simulink model "exact_linearization_new"  (R2021b)
settings: Solver=ode45  StartTime=0.0  StopTime=100.0  RelTol=1e-10
values from neighbouring files (symbols this model uses):
  G = 9.81    [edda.m]
  K0 = 1    [edda.m]
  K1 = 1    [edda.m]
  O1 = 3.1    [edda.m]
  O2 = 9.5    [edda.m]
  O3 = 0.24    [edda.m]
  O4 = 0.77    [edda.m]
settings Model: Creator=mbober  LastModifiedBy=mbober
settings DebuggingCC: UnderSpecifiedDimensionMsg=error

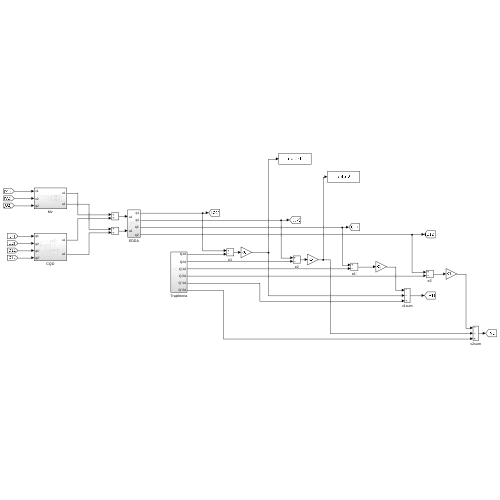
[thumbnail: Simulink's stored preview of the top-level diagram]
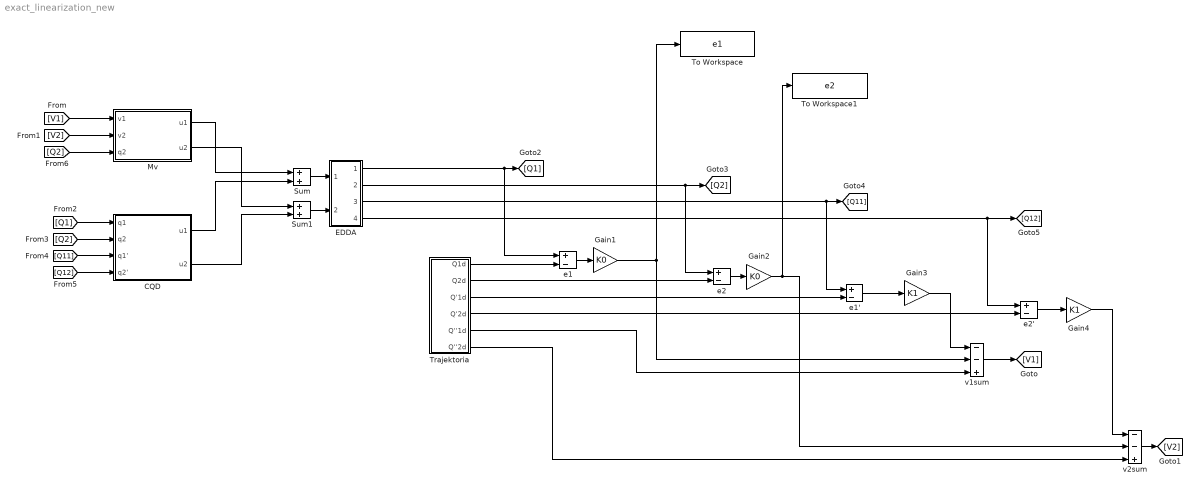
== system exact_linearization_new ==
  CQD : Subsystem
  EDDA : Subsystem
  Gain1 : Gain  Gain=K0
  Gain2 : Gain  Gain=K0
  Gain3 : Gain  Gain=K1
  Gain4 : Gain  Gain=K1
  Mv : Subsystem
  Sum : Sum
  Sum1 : Sum
  To Workspace : ToWorkspace  VariableName=e1  SampleTime=-1
  To Workspace1 : ToWorkspace  VariableName=e2  SampleTime=-1
  Trajektoria : Subsystem
  e1 : Sum  Inputs=+-
  e1' : Sum  Inputs=+-
  e2 : Sum  Inputs=+-
  e2' : Sum  Inputs=+-
  v1sum : Sum  Inputs=--+
  v2sum : Sum  Inputs=--+
  wires:
  Trajektoria/1(Q1d) -> e1/2
  EDDA/1(q1) -> [Q1], e1/1
  EDDA/2(q2) -> [Q2], e2/1
  Trajektoria/2(Q2d) -> e2/2
  EDDA/3(q1') -> [Q11], e1'/1
  Trajektoria/3(Q'1d) -> e1'/2
  EDDA/4(q2') -> e2'/1, [Q12]
  Trajektoria/4(Q'2d) -> e2'/2
  e1/1 -> Gain1/1
  e2/1 -> Gain2/1
  e1'/1 -> Gain3/1
  e2'/1 -> Gain4/1
  Gain3/1 -> v1sum/1
  Gain1/1 -> To Workspace/1, v1sum/2
  Gain4/1 -> v2sum/1
  Gain2/1 -> To Workspace1/1, v2sum/2
  Trajektoria/5(Q''1d) -> v1sum/3
  Trajektoria/6(Q''2d) -> v2sum/3
  v1sum/1 -> [V1]
  v2sum/1 -> [V2]
  [V1] -> Mv/1(v1)
  [V2] -> Mv/2(v2)
  [Q11] -> CQD/3(q1')
  [Q12] -> CQD/4(q2')
  [Q2] -> CQD/2(q2)
  [Q1] -> CQD/1(q1)
  [Q2] -> Mv/3(q2)
  Sum/1 -> EDDA/1(u1)
  Sum1/1 -> EDDA/2(u2)
  CQD/2(u2) -> Sum1/2
  Mv/2(u2) -> Sum1/1
  CQD/1(u1) -> Sum/2
  Mv/1(u1) -> Sum/1

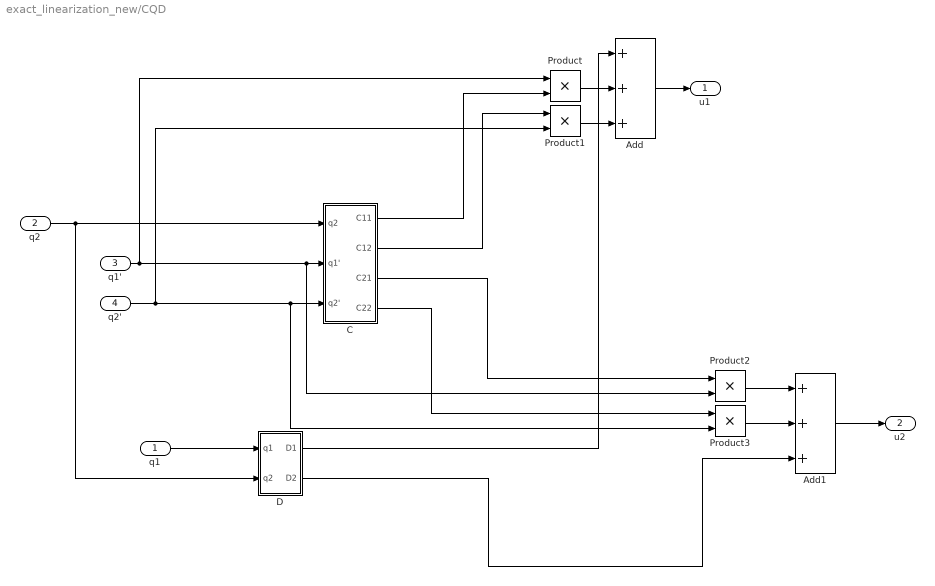
== system exact_linearization_new/CQD ==
  q1 : Inport
  q2 : Inport  Port=2
  q1' : Inport  Port=3
  q2' : Inport  Port=4
  Add : Sum  Inputs=+++
  Add1 : Sum  Inputs=+++
  C : Subsystem
  D : Subsystem
  Product{,1..3} (4 alike) : Product
  u1 : Outport
  u2 : Outport  Port=2
  wires:
  q2'/1 -> Product1/2, Product3/2, C/3(q2')
  q1'/1 -> Product2/2, C/2(q1'), Product/1
  q1/1 -> D/1(q1)
  q2/1 -> C/1(q2), D/2(q2)
  C/1(C11) -> Product/2
  C/2(C12) -> Product1/1
  Product/1 -> Add/2
  Product1/1 -> Add/3
  D/1(D1) -> Add/1
  Product3/1 -> Add1/2
  Product2/1 -> Add1/1
  D/2(D2) -> Add1/3
  C/3(C21) -> Product2/1
  C/4(C22) -> Product3/1
  Add/1 -> u1/1
  Add1/1 -> u2/1

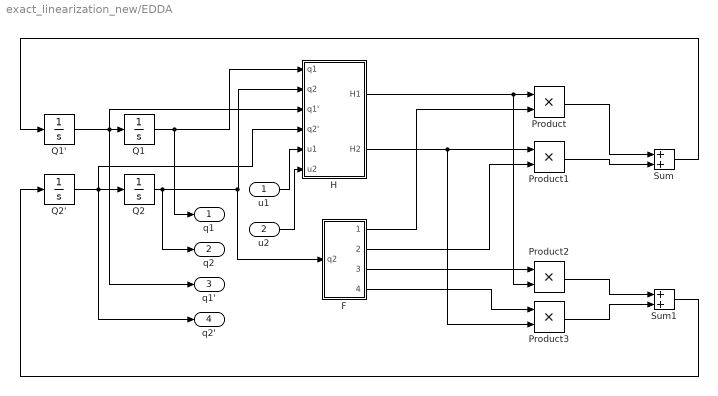
== system exact_linearization_new/EDDA ==
  u1 : Inport
  u2 : Inport  Port=2
  F : Subsystem
  H : Subsystem
  Product{,1..3} (4 alike) : Product
  Q1 : Integrator
  Q1' : Integrator
  Q2 : Integrator
  Q2' : Integrator
  Sum : Sum
  Sum1 : Sum
  q1 : Outport
  q2 : Outport  Port=2
  q1' : Outport  Port=3
  q2' : Outport  Port=4
  wires:
  Sum/1 -> Q1'/1
  F/3(F21) -> Product2/1
  u1/1 -> H/5(u1)
  Q2/1 -> q2/1, F/1(q2), H/2(q2)
  F/1(F11) -> Product/2
  Q1'/1 -> q1'/1, H/3(q1'), Q1/1
  Product1/1 -> Sum/2
  Q1/1 -> q1/1, H/1(q1)
  Q2'/1 -> q2'/1, H/4(q2'), Q2/1
  H/2(H2) -> Product3/2, Product1/1
  F/2(F12) -> Product1/2
  Sum1/1 -> Q2'/1
  u2/1 -> H/6(u2)
  H/1(H1) -> Product2/2, Product/1
  Product/1 -> Sum/1
  Product2/1 -> Sum1/1
  Product3/1 -> Sum1/2
  F/4(F22) -> Product3/1

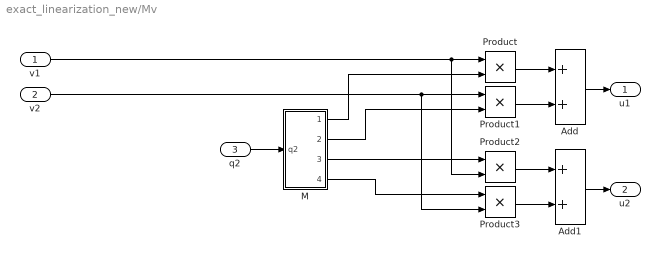
== system exact_linearization_new/Mv ==
  v1 : Inport
  v2 : Inport  Port=2
  q2 : Inport  Port=3
  Add : Sum
  Add1 : Sum
  M : Subsystem
  Product{,1..3} (4 alike) : Product
  u1 : Outport
  u2 : Outport  Port=2
  wires:
  q2/1 -> M/1(q2)
  Add/1 -> u1/1
  M/1(M11) -> Product/2
  v1/1 -> Product2/2, Product/1
  M/2(M12) -> Product1/2
  v2/1 -> Product3/2, Product1/1
  M/3(M21) -> Product2/1
  M/4(M22) -> Product3/1
  Product1/1 -> Add/2
  Product/1 -> Add/1
  Product2/1 -> Add1/1
  Product3/1 -> Add1/2
  Add1/1 -> u2/1

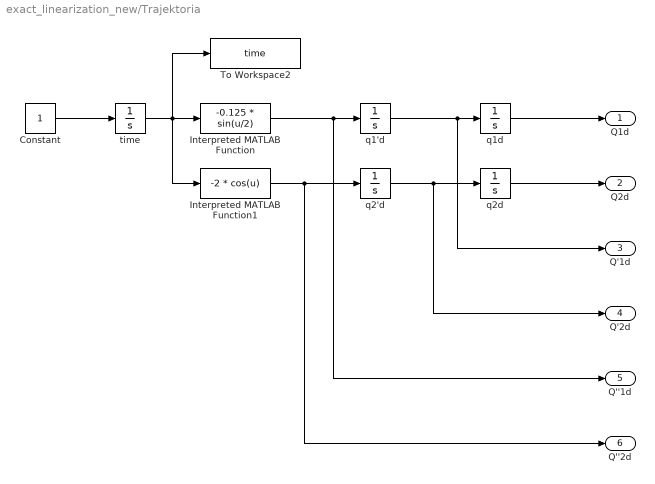
== system exact_linearization_new/Trajektoria ==
  Constant : Constant
  Interpreted MATLAB Function : MATLABFcn  MATLABFcn=-0.125 * sin(u/2)
  Interpreted MATLAB Function1 : MATLABFcn  MATLABFcn=-2 * cos(u)
  To Workspace2 : ToWorkspace  VariableName=time  SampleTime=-1
  q1'd : Integrator  InitialCondition=0.25
  q1d : Integrator
  q2'd : Integrator
  q2d : Integrator  InitialCondition=2
  time : Integrator
  Q1d : Outport
  Q2d : Outport  Port=2
  Q'1d : Outport  Port=3
  Q'2d : Outport  Port=4
  Q''1d : Outport  Port=5
  Q''2d : Outport  Port=6
  wires:
  q1d/1 -> Q1d/1
  Interpreted MATLAB Function/1 -> Q''1d/1, q1'd/1
  q2d/1 -> Q2d/1
  Interpreted MATLAB Function1/1 -> Q''2d/1, q2'd/1
  q1'd/1 -> Q'1d/1, q1d/1
  q2'd/1 -> Q'2d/1, q2d/1
  Constant/1 -> time/1
  time/1 -> Interpreted MATLAB Function1/1, To Workspace2/1, Interpreted MATLAB Function/1

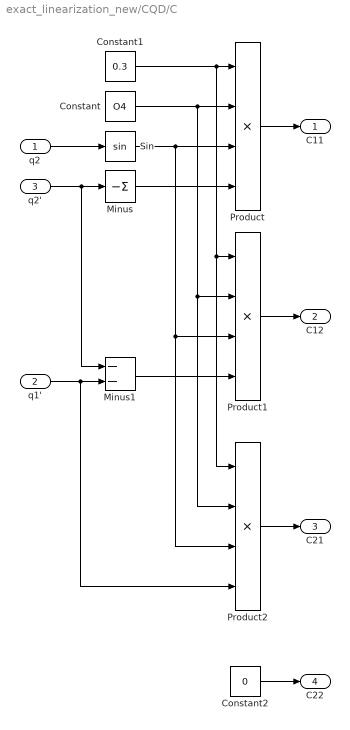
== system exact_linearization_new/CQD/C ==
  q2 : Inport
  q1' : Inport  Port=2
  q2' : Inport  Port=3
  Constant : Constant  Value=O4
  Constant1 : Constant  Value=0.3
  Constant2 : Constant  Value=0
  Minus : Sum  Inputs=-
  Minus1 : Sum  Inputs=--
  Product : Product  Inputs=4
  Product1 : Product  Inputs=4
  Product2 : Product  Inputs=4
  Sin : Trigonometry
  C11 : Outport
  C12 : Outport  Port=2
  C21 : Outport  Port=3
  C22 : Outport  Port=4
  wires:
  q2/1 -> Sin/1
  Sin/1 -> Product2/3, Product1/3, Product/3
  Constant/1 -> Product2/2, Product1/2, Product/2
  Constant1/1 -> Product2/1, Product1/1, Product/1
  Product/1 -> C11/1
  Minus/1 -> Product/4
  q2'/1 -> Minus1/1, Minus/1
  Minus1/1 -> Product1/4
  q1'/1 -> Product2/4, Minus1/2
  Product1/1 -> C12/1
  Product2/1 -> C21/1
  Constant2/1 -> C22/1

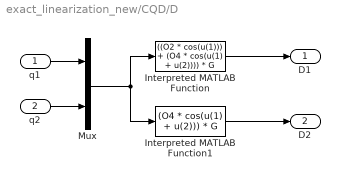
== system exact_linearization_new/CQD/D ==
  q1 : Inport
  q2 : Inport  Port=2
  Interpreted MATLAB Function : MATLABFcn  MATLABFcn=((O2 * cos(u(1))) + (O4 * cos(u(1) + u(2)))) * G
  Interpreted MATLAB Function1 : MATLABFcn  MATLABFcn=(O4 * cos(u(1) + u(2))) * G
  Mux : Mux  Inputs=2
  D1 : Outport
  D2 : Outport  Port=2
  wires:
  Interpreted MATLAB Function1/1 -> D2/1
  q1/1 -> Mux/1
  Mux/1 -> Interpreted MATLAB Function/1, Interpreted MATLAB Function1/1
  q2/1 -> Mux/2
  Interpreted MATLAB Function/1 -> D1/1

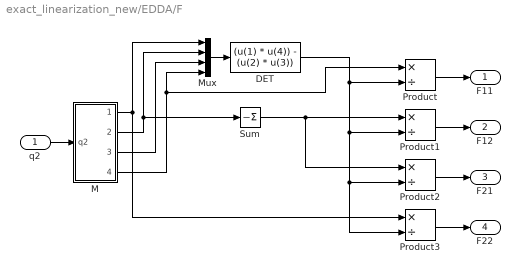
== system exact_linearization_new/EDDA/F ==
  q2 : Inport
  DET : MATLABFcn  MATLABFcn=(u(1) * u(4)) - (u(2) * u(3))  OutputDimensions=1
  M : Subsystem
  Mux : Mux
  Product{,1..3} (4 alike) : Product  Inputs=*/
  Sum : Sum  Inputs=-
  F11 : Outport
  F12 : Outport  Port=2
  F21 : Outport  Port=3
  F22 : Outport  Port=4
  wires:
  Product1/1 -> F12/1
  Mux/1 -> DET/1
  Product2/1 -> F21/1
  Product/1 -> F11/1
  M/2(M12) -> Mux/2, Sum/1
  M/1(M11) -> Product3/1, Mux/1
  M/4(M22) -> Product/1, Mux/4
  DET/1 -> Product/2, Product2/2, Product3/2, Product1/2
  Product3/1 -> F22/1
  q2/1 -> M/1(q2)
  M/3(M21) -> Mux/3
  Sum/1 -> Product2/1, Product1/1

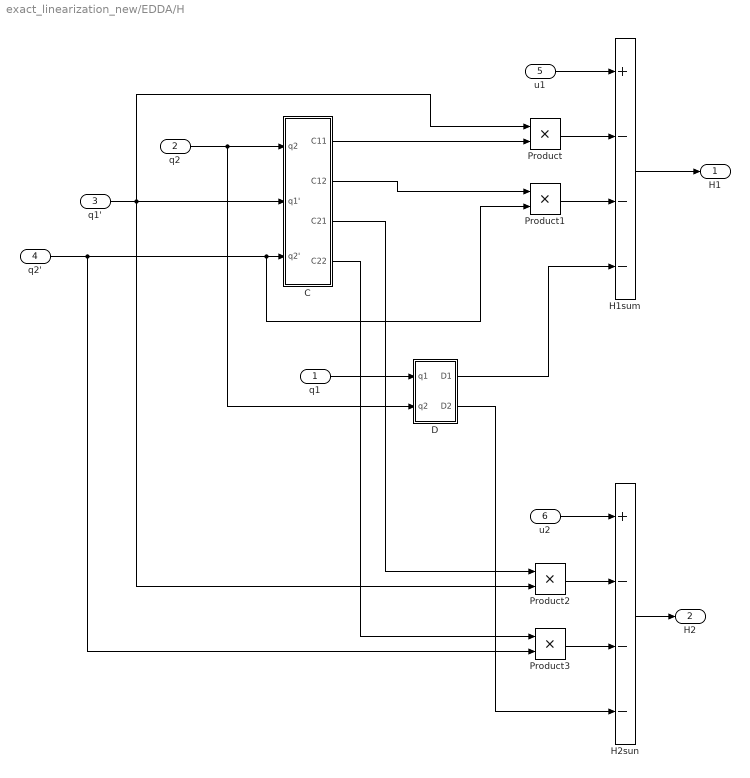
== system exact_linearization_new/EDDA/H ==
  q1 : Inport
  q2 : Inport  Port=2
  q1' : Inport  Port=3
  q2' : Inport  Port=4
  u1 : Inport  Port=5
  u2 : Inport  Port=6
  C : Subsystem
  D : Subsystem
  H1sum : Sum  Inputs=+---  OutMin=[1]  OutMax=[1]
  H2sun : Sum  Inputs=+---
  Product{,1..3} (4 alike) : Product
  H1 : Outport
  H2 : Outport  Port=2
  wires:
  Product2/1 -> H2sun/2
  C/4(C22) -> Product3/1
  Product1/1 -> H1sum/3
  D/1(D1) -> H1sum/4
  q1'/1 -> C/2(q1'), Product/1, Product2/2
  Product/1 -> H1sum/2
  q1/1 -> D/1(q1)
  q2/1 -> D/2(q2), C/1(q2)
  C/1(C11) -> Product/2
  u2/1 -> H2sun/1
  C/3(C21) -> Product2/1
  C/2(C12) -> Product1/1
  H1sum/1 -> H1/1
  D/2(D2) -> H2sun/4
  H2sun/1 -> H2/1
  Product3/1 -> H2sun/3
  q2'/1 -> Product1/2, C/3(q2'), Product3/2
  u1/1 -> H1sum/1

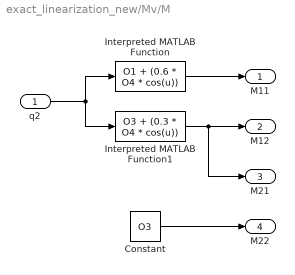
== system exact_linearization_new/Mv/M ==
  q2 : Inport
  Constant : Constant  Value=O3
  Interpreted MATLAB Function : MATLABFcn  MATLABFcn=O1 + (0.6 * O4 * cos(u))
  Interpreted MATLAB Function1 : MATLABFcn  MATLABFcn=O3 + (0.3 * O4 * cos(u))
  M11 : Outport
  M12 : Outport  Port=2
  M21 : Outport  Port=3
  M22 : Outport  Port=4
  wires:
  Interpreted MATLAB Function/1 -> M11/1
  q2/1 -> Interpreted MATLAB Function1/1, Interpreted MATLAB Function/1
  Interpreted MATLAB Function1/1 -> M21/1, M12/1
  Constant/1 -> M22/1

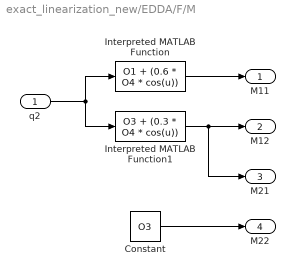
== system exact_linearization_new/EDDA/F/M ==
  q2 : Inport
  Constant : Constant  Value=O3
  Interpreted MATLAB Function : MATLABFcn  MATLABFcn=O1 + (0.6 * O4 * cos(u))
  Interpreted MATLAB Function1 : MATLABFcn  MATLABFcn=O3 + (0.3 * O4 * cos(u))
  M11 : Outport
  M12 : Outport  Port=2
  M21 : Outport  Port=3
  M22 : Outport  Port=4
  wires:
  Interpreted MATLAB Function/1 -> M11/1
  q2/1 -> Interpreted MATLAB Function1/1, Interpreted MATLAB Function/1
  Interpreted MATLAB Function1/1 -> M21/1, M12/1
  Constant/1 -> M22/1

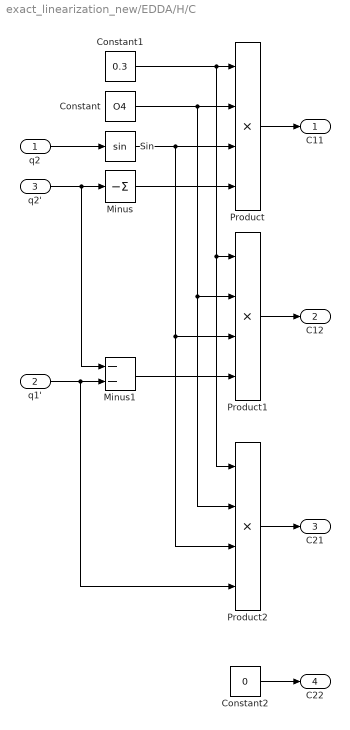
== system exact_linearization_new/EDDA/H/C ==
  q2 : Inport  OutMax=[1]
  q1' : Inport  Port=2  OutMax=[1]
  q2' : Inport  Port=3  OutMax=[1]
  Constant : Constant  Value=O4
  Constant1 : Constant  Value=0.3
  Constant2 : Constant  Value=0
  Minus : Sum  Inputs=-
  Minus1 : Sum  Inputs=--
  Product : Product  Inputs=4
  Product1 : Product  Inputs=4
  Product2 : Product  Inputs=4
  Sin : Trigonometry
  C11 : Outport  OutMax=[1]
  C12 : Outport  Port=2  OutMax=[1]
  C21 : Outport  Port=3  OutMax=[1]
  C22 : Outport  Port=4  OutMax=[1]
  wires:
  q2/1 -> Sin/1
  Sin/1 -> Product2/3, Product1/3, Product/3
  Constant/1 -> Product2/2, Product1/2, Product/2
  Constant1/1 -> Product2/1, Product1/1, Product/1
  Product/1 -> C11/1
  Minus/1 -> Product/4
  q2'/1 -> Minus1/1, Minus/1
  Minus1/1 -> Product1/4
  q1'/1 -> Product2/4, Minus1/2
  Product1/1 -> C12/1
  Product2/1 -> C21/1
  Constant2/1 -> C22/1

== system exact_linearization_new/EDDA/H/D ==
  q1 : Inport  OutMin=[1]  OutMax=[1]
  q2 : Inport  Port=2  OutMin=[1]  OutMax=[1]
  Interpreted MATLAB Function : MATLABFcn  MATLABFcn=((O2 * cos(u(1))) + (O4 * cos(u(1) + u(2)))) * G  OutputDimensions=1
  Interpreted MATLAB Function1 : MATLABFcn  MATLABFcn=(O4 * cos(u(1) + u(2))) * G  OutputDimensions=1
  Mux : Mux  Inputs=2
  D1 : Outport  OutMax=[1]
  D2 : Outport  Port=2  OutMax=[1]
  wires:
  Interpreted MATLAB Function1/1 -> D2/1
  q1/1 -> Mux/1
  Mux/1 -> Interpreted MATLAB Function/1, Interpreted MATLAB Function1/1
  q2/1 -> Mux/2
  Interpreted MATLAB Function/1 -> D1/1
